simulink model "ex_2"  (R2023b)
settings: Solver=VariableStepAuto  StartTime=0.0  StopTime=10.0  RelTol=1e-3
settings Model: Creator=LucasDaiPráMartens  LastModifiedBy=LucasDaiPráMartens

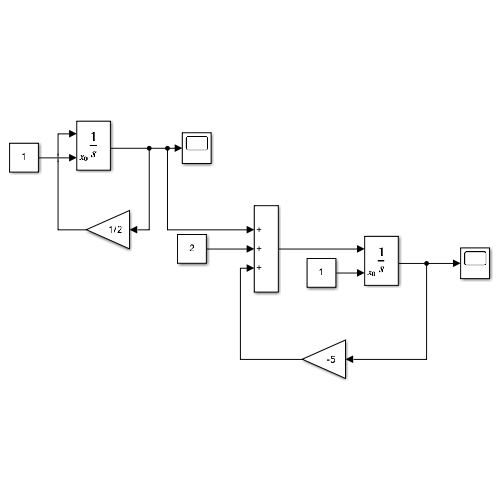
[thumbnail: Simulink's stored preview of the top-level diagram]
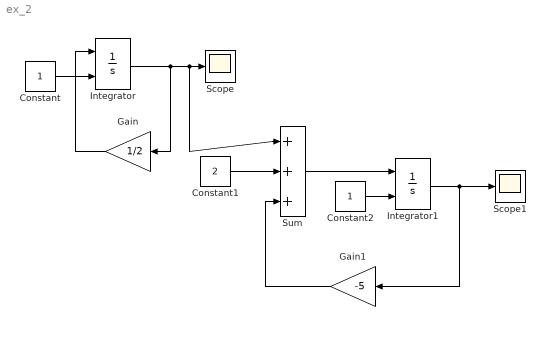
== system ex_2 ==
  Constant : Constant
  Constant1 : Constant  Value=2
  Constant2 : Constant
  Gain : Gain  Gain=1/2
  Gain1 : Gain  Gain=-5
  Integrator : Integrator  InitialConditionSource=external
  Integrator1 : Integrator  InitialConditionSource=external
  Scope : Scope
  Scope1 : Scope
  Sum : Sum  Inputs=|+|+|+|
  wires:
  Integrator/1 -> Gain/1, Sum/1, Scope/1
  Gain/1 -> Integrator/1
  Constant/1 -> Integrator/2
  Constant1/1 -> Sum/2
  Sum/1 -> Integrator1/1
  Constant2/1 -> Integrator1/2
  Integrator1/1 -> Gain1/1, Scope1/1
  Gain1/1 -> Sum/3
